simulink model "Validazione_cascata"  (R2023b)
settings: Solver=VariableStepAuto  StartTime=0.0  StopTime=10.0  RelTol=1e-3
values from neighbouring files (symbols this model uses):
  den_mag_C2 = Gden{1}    [Controllo_un_anello_v2.m]    (also in Controllore_testato.m; controllo_un_anello.m)
  Lower_bound_V = -23    [Controllo_un_anello_v2.m]    (also in Controllore_testato.m = 0; controllo_un_anello.m; controllore_piu_anelli.m)
  num_mag_C2 = Gnum{1}    [Controllo_un_anello_v2.m]    (also in Controllore_testato.m; controllo_un_anello.m)
  Upper_bound_V = 23    [Controllo_un_anello_v2.m]    (also in Controllore_testato.m; controllo_un_anello.m; controllore_piu_anelli.m)
undefined symbols (not defined in the file or in its folder): ki2, kp2, Lc, Rtot
libraries: slpidlib x1
settings Model: Creator=lollo  LastModifiedBy=lollo

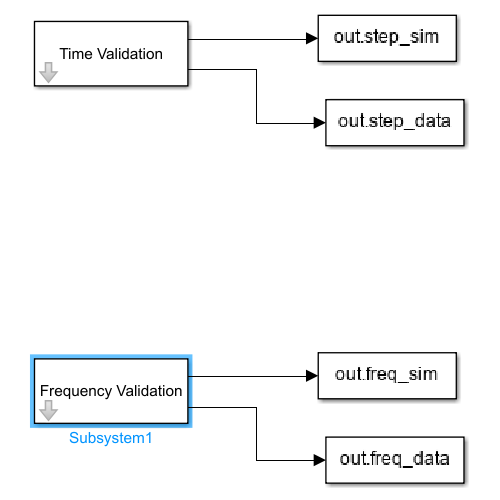
[thumbnail: Simulink's stored preview of the top-level diagram]
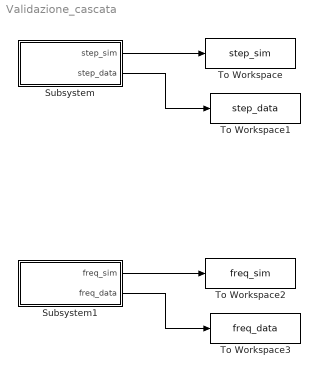
== system Validazione_cascata ==
  Subsystem : Subsystem
      mask DialogControl DescGroupVar Prompt: Time Validation
      mask DialogControl DescTextVar Prompt: Questo Subsystem serve per la validazione nel TEMPO del controllore in cascata
      mask Display: disp('Time Validation')
  Subsystem1 : Subsystem
      mask DialogControl DescGroupVar Prompt: Frequency Validation
      mask DialogControl DescTextVar Prompt: Questo Subsystem serve per la validazione in FREQUENZA del controllore in cascata
      mask Display: disp('Frequency Validation')
  To Workspace : ToWorkspace  VariableName=step_sim  SaveFormat=Timeseries  SampleTime=-1
  To Workspace1 : ToWorkspace  VariableName=step_data  SaveFormat=Timeseries  SampleTime=-1
  To Workspace2 : ToWorkspace  VariableName=freq_sim  SaveFormat=Timeseries  SampleTime=-1
  To Workspace3 : ToWorkspace  VariableName=freq_data  SaveFormat=Timeseries  SampleTime=-1
  wires:
  Subsystem/1(step_sim) -> To Workspace/1
  Subsystem/2(step_data) -> To Workspace1/1
  Subsystem1/1(freq_sim) -> To Workspace2/1
  Subsystem1/2(freq_data) -> To Workspace3/1

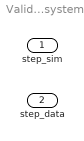
== system Validazione_cascata/Subsystem ==
  step_sim : Outport
  step_data : Outport  Port=2

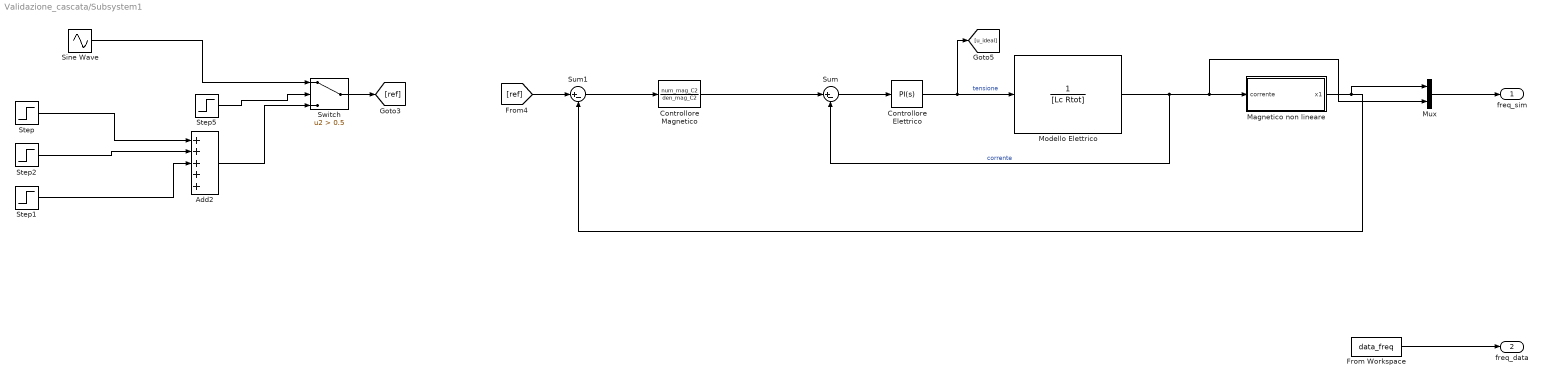
== system Validazione_cascata/Subsystem1 ==
  Add2 : Sum  Inputs=+++++
  Controllore Elettrico : slpidlib/PID Controller  Controller=PI  Form=Parallel  TimeDomain=Continuous-time  UseExternalTs=off  SampleTime=-1  IntegratorMethod=Forward Euler  FilterMethod=Forward Euler  ControllerParametersSource=internal  P=kp2  I=ki2  UseKiTs=off  D=0  N=100  UseFilter=on  TunerSelectOption=Transfer Function Based (PID Tuner App)  InitialConditionSource=internal  InitialConditionForIntegrator=0  InitialConditionForFilter=0  DifferentiatorICPrevScaledInput=0  ExternalReset=none  TrackingMode=off  Kt=1  LimitOutput=on  SatLimitsSource=internal  UpperSaturationLimit=Upper_bound_V  LowerSaturationLimit=Lower_bound_V  LinearizeAsGain=on  AntiWindupMode=none  Kb=1  LimitIntegrator=off  UpperIntegratorSaturationLimit=inf  LowerIntegratorSaturationLimit=-inf  POutMin=[]  POutMax=[]  IOutMin=[]  IOutMax=[]  DOutMin=[]  DOutMax=[]  NOutMin=[]  NOutMax=[]  SumOutMin=[]  SumOutMax=[]  SaturationOutMin=[]  SaturationOutMax=[]  PParamMin=[]  PParamMax=[]  IParamMin=[]  IParamMax=[]  DParamMin=[]  DParamMax=[]  NParamMin=[]  NParamMax=[]  KbParamMin=[]  KbParamMax=[]  KtParamMin=[]  KtParamMax=[]  KbOutMin=[]  KbOutMax=[]  KtOutMin=[]  KtOutMax=[]  IntegratorOutMin=[]  IntegratorOutMax=[]  FilterOutMin=[]  FilterOutMax=[]  SumI1OutMin=[]  SumI1OutMax=[]  SumI2OutMin=[]  SumI2OutMax=[]  SumI3OutMin=[]  SumI3OutMax=[]  SumI4OutMin=[]  SumI4OutMax=[]  SumDOutMin=[]  SumDOutMax=[]  DifferentiatorOutMin=[]  DifferentiatorOutMax=[]  FilterDiffOutCoefMin=[]  FilterDiffOutCoefMax=[]  ReciprocalOutMin=[]  ReciprocalOutMax=[]  SumDenOutMin=[]  SumDenOutMax=[]  SumNumOutMin=[]  SumNumOutMax=[]  DivideOutMin=[]  DivideOutMax=[]  UdiffTsProdOutMin=[]  UdiffTsProdOutMax=[]  NTsProdOutMin=[]  NTsProdOutMax=[]  UintegralTsProdOutMin=[]  UintegralTsProdOutMax=[]  UngainTsProdOutMin=[]  UngainTsProdOutMax=[]  ClampingZeroOutDataTypeStr=Inherit: Inherit via back propagation  ClampingZeroOutMin=[]  ClampingZeroOutMax=[]  FilterDenConstantOutDataTypeStr=Inherit: Inherit via back propagation  FilterDenConstantOutMin=[]  FilterDenConstantOutMax=[]  PCopyOutDataTypeStr=Inherit: Inherit via back propagation  PCopyOutMin=[]  PCopyOutMax=[]  NCopyOutDataTypeStr=Inherit: Inherit via back propagation  NCopyOutMin=[]  NCopyOutMax=[]  IntegratorContinuousStateAttributes=''  IntegratorStateMustResolveToSignalObject=off  IntegratorRTWStateStorageClass=Auto  FilterContinuousStateAttributes=''  FilterStateMustResolveToSignalObject=off  FilterRTWStateStorageClass=Auto  ParallelPVariant=InternalParameters  IdealPVariant=Disabled  IVariant=InternalParameters  DVariant=Disabled  IntegratorVariant=Continuous  SatVariant=Enabled  AWVariant=Passthrough  PCopyVariant=Disabled  TRVariant=Disabled  FdbkBlocksVariant=Forward  IdealPFdbkVariant=Disabled  SatFdbkVariant=Disabled  DerivativeFilterVariant=Disabled  NVariant=Disabled  NCopyVariant=Disabled_SignalSpec  FilterICVariant=Disabled  IntegratorICVariant=InternalICs  ExternalResetVariant=Disabled  TRSumVariant=Passthrough  SumFdbkVariant=Disabled  SumVariant=Sum_PI  TsampFilterVariant=InternalTs  TsampNgainVariant=Passthrough  TsampIntegralVariant=Disabled_SignalSpec  ExternalSaturationOutDataTypeStr=Inherit: Same as second input
  Controllore Magnetico : TransferFcn  Numerator=num_mag_C2  Denominator=den_mag_C2
  From Workspace : FromWorkspace  VariableName=data_freq
  Magnetico non lineare : Subsystem
  Modello Elettrico : TransferFcn  Denominator=[Lc Rtot]
  Mux : Mux  Inputs=2
  Sine Wave : Sin  Amplitude=0.0001  Bias=0.003  Frequency=110  Phase=2.2566  SampleTime=0
  Step : Step  Time=0  After=0.001  SampleTime=0
  Step1 : Step  Time=2  After=0.001  SampleTime=0
  Step2 : Step  Time=5  After=0.001  SampleTime=0
  Step5 : Step  Time=7  SampleTime=0
  Sum : Sum  Inputs=|+-
  Sum1 : Sum  Inputs=|+-
  Switch : Switch  Criteria=u2 > Threshold  Threshold=0.5  SaturateOnIntegerOverflow=off  InputSameDT=off
  freq_sim : Outport
  freq_data : Outport  Port=2
  wires:
  Switch/1 -> [ref]
  Step5/1 -> Switch/2
  Step1/1 -> Add2/3
  Add2/1 -> Switch/3
  Sine Wave/1 -> Switch/1
  Step/1 -> Add2/1
  Step2/1 -> Add2/2
  [ref] -> Sum1/1
  Sum1/1 -> Controllore Magnetico/1
  Sum/1 -> Controllore Elettrico/1
  Modello Elettrico/1 -> Sum/2, Mux/2, Magnetico non lineare/1(corrente)  "corrente"
  Magnetico non lineare/1(x1) -> Mux/1, Sum1/2
  Controllore Elettrico/1 -> [u_ideal], Modello Elettrico/1  "tensione"
  Controllore Magnetico/1 -> Sum/1
  Mux/1 -> freq_sim/1
  From Workspace/1 -> freq_data/1

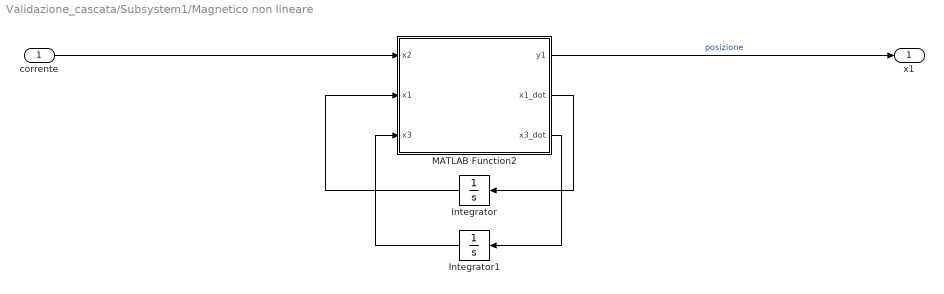
== system Validazione_cascata/Subsystem1/Magnetico non lineare ==
  corrente : Inport
  Integrator : Integrator
  Integrator1 : Integrator
  MATLAB Function2 : MATLAB Function  TreatAsAtomicUnit=on
  x1 : Outport
  wires:
  corrente/1 -> MATLAB Function2/1(x2)
  MATLAB Function2/1(y1) -> x1/1  "posizione"
  MATLAB Function2/2(x1_dot) -> Integrator/1
  Integrator/1 -> MATLAB Function2/2(x1)
  MATLAB Function2/3(x3_dot) -> Integrator1/1
  Integrator1/1 -> MATLAB Function2/3(x3)

== matlab function Validazione_cascata/Subsystem1/Magnetico non lineare/MATLAB Function2 ==
  data: y1 output; x2 input; x1_dot output; x1 input; x3 input; x3_dot output
function [y1,x1_dot, x3_dot] = fcn(x2, x1, x3)
    m = 0.0657;
    g = 9.81;
    k_mag = 2.4405e-05;
    Rtot = 9.7585;
    Lc = 0.3708;
    y0 = 0.012;
    
    x1_dot = x3;
    if x1 < y0
        x3_dot = (k_mag/m)*(x2/(y0-x1))^2 - g;
    else
        x1 = 0.012;
        x3_dot = 0;
        x3 = 0;
    end

    
    % condizioni
    if x1 <=0 && x3_dot < 0
        x1 = 0;
        x3 = 0;
        x3_dot = 0;
    end
y1 = x1;
